simulink model "pd_plus_testings_7DOF"  (R2022b)
settings: Solver=VariableStepAuto  StartTime=0.0  StopTime=101  RelTol=1e-3
InitFcn:
  | parameters_7dof;
undefined symbols (not defined in the file): param_robot, q_0
settings Model: Creator=emu  LastModifiedBy=emu

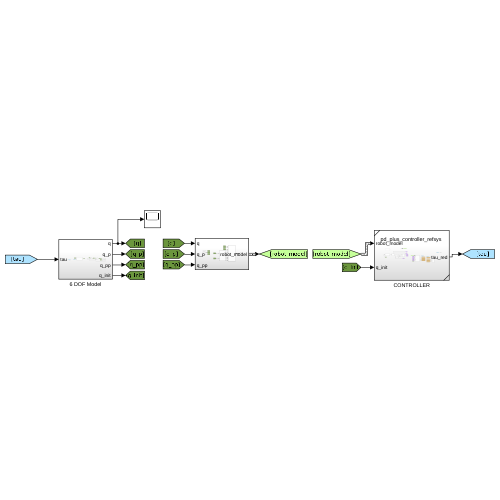
[thumbnail: Simulink's stored preview of the top-level diagram]
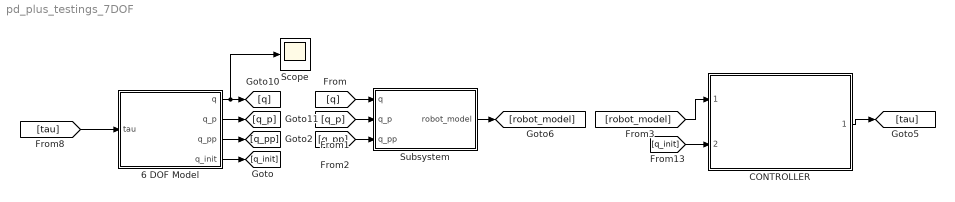
== system pd_plus_testings_7DOF ==
  6 DOF Model : Subsystem
  CONTROLLER : Subsystem  ReferencedSubsystem=pd_plus_controller_refsys
  Scope : Scope
  Subsystem : Subsystem
  wires:
  [q] -> Subsystem/1(q)
  [q_pp] -> Subsystem/3(q_pp)
  [q_p] -> Subsystem/2(q_p)
  [robot_model] -> CONTROLLER/1
  6 DOF Model/1(q) -> Scope/1, [q]
  6 DOF Model/2(q_p) -> [q_p]
  6 DOF Model/3(q_pp) -> [q_pp]
  [tau] -> 6 DOF Model/1(tau)
  Subsystem/1(robot_model) -> [robot_model]
  CONTROLLER/1 -> [tau]
  [q_init] -> CONTROLLER/2
  6 DOF Model/4(q_init) -> [q_init]

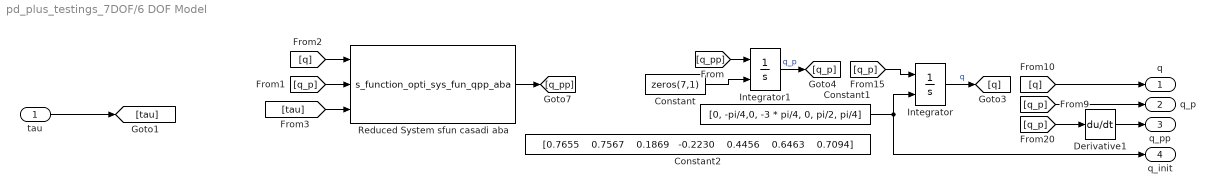
== system pd_plus_testings_7DOF/6 DOF Model ==
  tau : Inport
  Constant : Constant  Value=zeros(7,1)
  Constant1 : Constant  Value=[0, -pi/4,0, -3 * pi/4, 0, pi/2, pi/4]
  Constant2 : Constant  Value="[0.7655    0.7567    0.1869   -0.2230    0.4456    0.6463    0.7094]"
  Derivative1 : Derivative
  Integrator : Integrator  InitialConditionSource=external  InitialCondition=q_0  UpperSaturationLimit=param_robot.q_limit_upper  LowerSaturationLimit=param_robot.q_limit_lower
  Integrator1 : Integrator  InitialConditionSource=external  InitialCondition=param_robot.q_0_p_ref  UpperSaturationLimit=param_robot.q_p_limit_upper  LowerSaturationLimit=param_robot.q_p_limit_lower
  Reduced System sfun casadi aba : S-Function  FunctionName=s_function_opti_sys_fun_qpp_aba  SFunctionModules='sys_fun_qpp_aba'  SFunctionDeploymentMode=off  EnableBusSupport=off
  q : Outport
  q_p : Outport  Port=2
  q_pp : Outport  Port=3
  q_init : Outport  Port=4
  wires:
  [q_p] -> Derivative1/1
  Derivative1/1 -> q_pp/1
  tau/1 -> [tau]
  [q_p] -> q_p/1
  [q_p] -> Integrator/1
  Integrator1/1 -> [q_p]  "q_p"
  Integrator/1 -> [q]  "q"
  [q] -> q/1
  [q_pp] -> Integrator1/1
  Constant/1 -> Integrator1/2
  Constant1/1 -> q_init/1, Integrator/2
  Reduced System sfun casadi aba/1 -> [q_pp]
  [q_p] -> Reduced System sfun casadi aba/2
  [q] -> Reduced System sfun casadi aba/1
  [tau] -> Reduced System sfun casadi aba/3

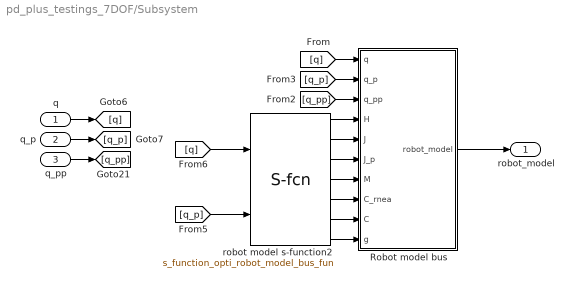
== system pd_plus_testings_7DOF/Subsystem ==
  q : Inport
  q_p : Inport  Port=2
  q_pp : Inport  Port=3
  Robot model bus : MATLAB Function  TreatAsAtomicUnit=on
  robot model s-function2 : S-Function  FunctionName=s_function_opti_robot_model_bus_fun  SFunctionModules='robot_model_bus_fun'  SFunctionDeploymentMode=off  EnableBusSupport=off
  robot_model : Outport  OutDataTypeStr=Bus: robot_model
  wires:
  q_pp/1 -> [q_pp]
  q_p/1 -> [q_p]
  q/1 -> [q]
  robot model s-function2/2 -> Robot model bus/5(J)
  [q] -> robot model s-function2/1
  Robot model bus/1(robot_model) -> robot_model/1
  robot model s-function2/5 -> Robot model bus/8(C_rnea)
  robot model s-function2/4 -> Robot model bus/7(M)
  [q_pp] -> Robot model bus/3(q_pp)
  robot model s-function2/6 -> Robot model bus/9(C)
  [q] -> Robot model bus/1(q)
  robot model s-function2/7 -> Robot model bus/10(g)
  [q_p] -> Robot model bus/2(q_p)
  robot model s-function2/3 -> Robot model bus/6(J_p)
  robot model s-function2/1 -> Robot model bus/4(H)
  [q_p] -> robot model s-function2/2

== matlab function pd_plus_testings_7DOF/Subsystem/Robot model bus ==
  settings: updateMethod=DISCRETE  sampleTime=param_global.Ta
  data: q input; q_p input; q_pp input; H input; J input; J_p input; M input; C_rnea input; C input; g input; robot_model output Bus: robot_model
function robot_model = fcn(q, q_p, q_pp, H, J, J_p, M, C_rnea, C, g)
% Parameters
robot_model=struct();
robot_model.q=q;                    % generalized coordinates
robot_model.q_p=q_p;                % time derivative of generalized coordinates
robot_model.q_pp=q_pp;
robot_model.H=H;
robot_model.J=J;
robot_model.J_p=J_p;
robot_model.M=M;
robot_model.C_rnea=C_rnea; % C_rnea(q, q_p) = C(q, q_p)q_p + g(q) = n(q, q_p)
robot_model.C=C;
robot_model.g=g;
end
